simulink model "ex1_s"  (R2020a)
settings: Solver=VariableStepAuto  StartTime=0.0  StopTime=10.0  RelTol=1e-3
values from neighbouring files (symbols this model uses):
  den_G11 = [0.6 1]    [ex1.m]
  den_G12 = [0.7 1]    [ex1.m]
  den_G21 = [0.9 1]    [ex1.m]
  den_G22 = [1.5 1]    [ex1.m]
  den_Gr1 = [1 0]    [ex1.m]
  den_Gr2 = [1 0]    [ex1.m]
  num_G11 = [2]    [ex1.m]
  num_G12 = [0.1]    [ex1.m]
  num_G21 = [0.4]    [ex1.m]
  num_G22 = [5]    [ex1.m]
  num_Gr1 = [0.7 2.38]    [ex1.m]

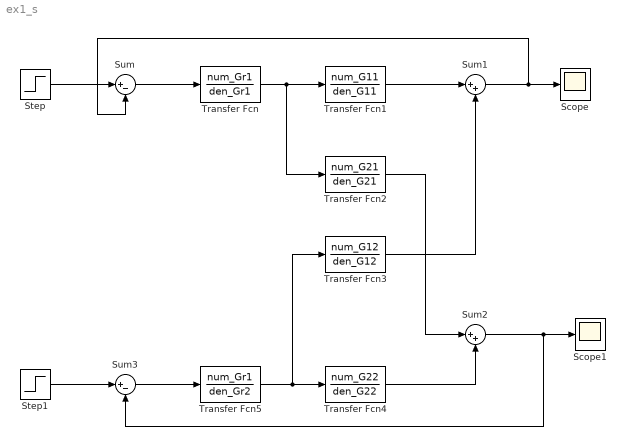
== system ex1_s ==
  Scope : Scope
  Scope1 : Scope
  Step : Step  SampleTime=0
  Step1 : Step  SampleTime=0
  Sum : Sum  Inputs=|+-
  Sum1 : Sum  Inputs=|++
  Sum2 : Sum  Inputs=|++
  Sum3 : Sum  Inputs=|+-
  Transfer Fcn : TransferFcn  Numerator=num_Gr1  Denominator=den_Gr1
  Transfer Fcn1 : TransferFcn  Numerator=num_G11  Denominator=den_G11
  Transfer Fcn2 : TransferFcn  Numerator=num_G21  Denominator=den_G21
  Transfer Fcn3 : TransferFcn  Numerator=num_G12  Denominator=den_G12
  Transfer Fcn4 : TransferFcn  Numerator=num_G22  Denominator=den_G22
  Transfer Fcn5 : TransferFcn  Numerator=num_Gr1  Denominator=den_Gr2
  wires:
  Step/1 -> Sum/1
  Sum/1 -> Transfer Fcn/1
  Transfer Fcn/1 -> Transfer Fcn2/1, Transfer Fcn1/1
  Transfer Fcn1/1 -> Sum1/1
  Sum1/1 -> Sum/2, Scope/1
  Transfer Fcn3/1 -> Sum1/2
  Transfer Fcn2/1 -> Sum2/1
  Transfer Fcn4/1 -> Sum2/2
  Transfer Fcn5/1 -> Transfer Fcn3/1, Transfer Fcn4/1
  Sum3/1 -> Transfer Fcn5/1
  Step1/1 -> Sum3/1
  Sum2/1 -> Sum3/2, Scope1/1
